simulink model "electrotac_feedback_emg"  (R2016b)
settings: Solver=FixedStepDiscrete  StartTime=0.0  StopTime=inf  FixedStep=0.02  RelTol=1e-3  EnableMultiTasking=on
undefined symbols (not defined in the file): DiscIntNeverNeededParam
libraries: PowermateLibrary x1, LIB_RehaMove3 x1, STIMYOLibrary x1
(part 1 of 3)
settings Model: SimulationMode=external  Creator=mendicus  LastModifiedBy=control
settings DataIOCC: LimitDataPoints=on  SaveFormat=Array  ReturnWorkspaceOutputs=on
settings OptimizationCC: LifeSpan=1
settings DebuggingCC: ReadBeforeWriteMsg=DisableAll  WriteAfterWriteMsg=DisableAll  WriteAfterReadMsg=DisableAll  SolverPrmCheckMsg=warning  MultiTaskDSMMsg=none  SFUnexpectedBacktrackingDiag=warning  SFNoUnconditionalDefaultTransitionDiag=warning  SFExecutionAtInitializationDiag=none
settings HardwareCC: ProdBitPerPointer=32  ProdBitPerSizeT=32  ProdBitPerPtrDiffT=32  ProdLargestAtomicFloat=None  ProdIntDivRoundTo=Undefined  ProdEndianess=Unspecified  ProdWordSize=32  ProdHWDeviceType=32-bit Generic
settings ModelReferenceCC: UpdateModelReferenceTargets=IfOutOfDate  PropagateSignalLabelsOutOfModel=off
settings SFSimCC: SFSimEcho=off
settings RTWCC: SystemTargetFile=ert_linux.tlc  MakeCommand=make_rtw OPTS=-DWITH_HW  TemplateMakefile=ert_linux.tmf  Description=Linux Embedded Coder  TargetLang=C++
settings CodeAppCC: IgnoreCustomStorageClasses=off
settings STFCustomTargetCC: ModelReferenceCompliant=off  CombineOutputUpdateFcns=on  ERTCustomFileBanners=on  SupportNonInlinedSFcns=off  RemoveResetFunc=on  SupportVariableSizeSignals=on  MATLABClassNameForMDSCustomization=Simulink.SoftwareTarget.ERTCustomization  GRTInterface=off  SystemTargetFile=ert_linux.tlc
settings ERTTargetCC: ModelReferenceCompliant=off  ParMdlRefBuildCompliant=off  CompOptLevelCompliant=off  ConcurrentExecutionCompliant=off  ERTFirstTimeCompliant=off  SupportContinuousTime=on  SupportVariableSizeSignals=on  ModelStepFunctionPrototypeControlCompliant=off  CPPClassGenCompliant=off  UseToolchainInfoCompliant=off  ExtMode=on  ERTCustomFileTemplate=ert_linux_file_process.tlc  ConvertIfToSwitch=off  SuppressUnreachableDefaultCases=off
settings ConfigComp: CovMetricSettings=dw  CovHtmlReporting=on  CovSaveCumulativeToWorkspaceVar=on  CovSaveSingleToWorkspaceVar=on  CovExternalEMLEnable=off  CovSFcnEnable=off

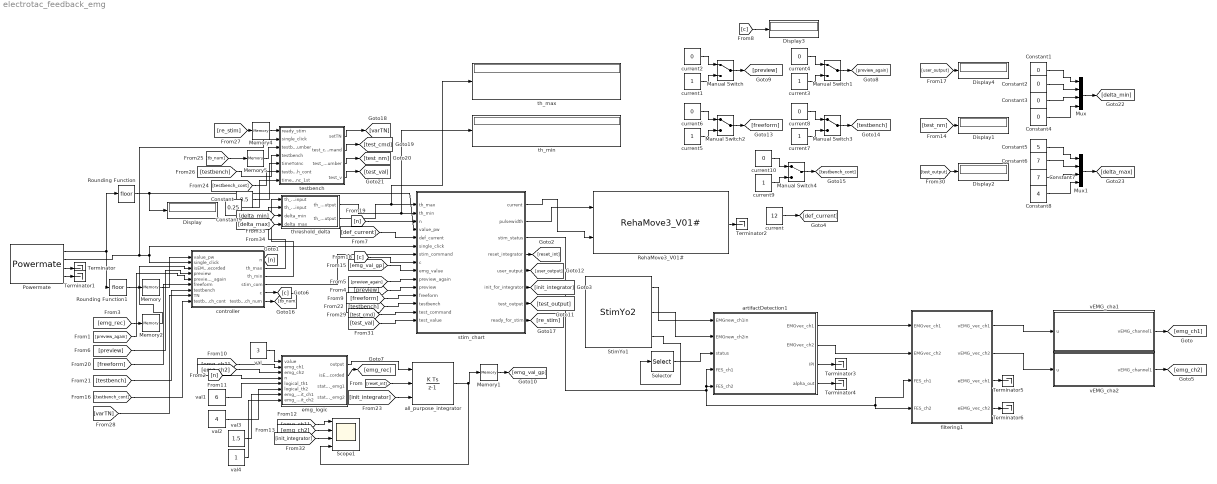
== system electrotac_feedback_emg ==
  Constant : Constant  Value=0.5
  Constant{1..4} (4 alike) : Constant  Value=0
  Constant5 : Constant  Value=5
  Constant6 : Constant  Value=7
  Constant7 : Constant  Value=7
  Constant8 : Constant  Value=4
  Constant9 : Constant  Value=0.25
  Display{,1..4} (5 alike) : Display
  Manual Switch{,1..4} (5 alike) : ManualSwitch
  Memory{,1..2,4..5} (5 alike) : Memory
  Mux : Mux
  Mux1 : Mux
  Powermate : PowermateLibrary/Powermate  pmin=0  pmax=1000  ptours=10  pstart=0  pbtnmode=0  pndoubleclick=50  Ts=0.02
  RehaMove3_V01# : LIB_RehaMove3/RehaMove3_V01#  stimDevicePath=/dev/ttyUSB0  stimChannels="[ 1  2  3  4 ]"  stimFrequency=50  stimRehaMoveProProtocol=Use the LowLevel protocol and use the user provieded pulse configs.  stimMaxCurrent=30  stimMaxPulsWidth=600  stimBlockID=STIM1  stimTextSampleTime=0.02s (based on stimulation frequency)  SampleTime=0.02  stimThreadInit=on  stimThreadData=on  stimAbortError=1  stimTestAgain=2  llPulseShape=0  llNumberOfParts=3  llMaxStimVoltage=120V  llActivateDenervation=off  mlFStim=0.5  mlFStimDynamic=off  mlFKeepAlive=1  mlUseSoftStart=off  mlUseRamps=off  mlRampsUpdates=1  mlRampsZeroUpdates=0  miscPrintBlockParam=on  miscPrintDeviceInfos=on  miscPrintSendInfos=on  miscPrintReceiveInfos=on  miscPrintInitInfos=on  miscPrintStimInfos=on  miscPrintRMPInitSettings=on  miscPrintSequenceErrors=on  miscPrintCorrectionChargeWarnings=on  miscPrintStats=on  miscUseColors=on  miscEnableAdvancedSettings=off  miscDisableVersionCheck=off
  Rounding Function : Rounding
  Rounding Function1 : Rounding
  Scope1 : Scope  NumInputPorts=4
  Selector : Selector  InputPortWidth=3  IndexOptions=Index vector (dialog)  Indices=[2]  OutputSizes=1
  StimYo1 : STIMYOLibrary/StimYo2  DeviceName='/dev/ttyUSB1'  frequency=4000  ch=[1 2]  vectorsize=200  syncmode=-1  ps_end=0  ss_start=0  ss_end=3  Ts=0.02
  Terminator{,1..6} (7 alike) : Terminator
  all_purpose_integrator : DiscreteIntegrator  ExternalReset=rising  InitialConditionSource=external  InitialConditionSetting=State (most efficient)  SampleTime=0.02  LimitOutput=on  UpperSaturationLimit=12  LowerSaturationLimit=0  ICPrevOutput=DiscIntNeverNeededParam  ICPrevScaledInput=DiscIntNeverNeededParam
  artifactDetection1 : MATLAB Function  TreatAsAtomicUnit=on  mask{emg_f_popup=4000, emg_f=4000, stim_f_popup=50, stim_f=50, L=80, peak_popup=MAD, complete=on, alpha_auto=on, alpha_init=3}
      mask prompts: emg_f_popup "EMG freq [Hz]"; emg_f "Value"; stim_f_popup "Stim freq [Hz]"; stim_f "Value"; peak_popup "Type"; complete "Last complete IPI"; alpha_auto "Automatic alpha"; alpha_init "Initial alpha"
      mask init:
      | alpha_in = [alpha_auto,alpha_init];
      | 
      | 
      | emg_ff = str2double(get_param(gcb,'emg_f'));
      | stim_ff = str2double(get_param(gcb,'stim_f'));
      | L = ceil(emg_f/stim_f);
      | assert(L <= 200, 'Maximum L = emg_f/stim_f is 200.');
  controller : Stateflow chart  TreatAsAtomicUnit=on
  current : Constant  Value=12
  current{1,3,5,7,9} (5 alike) : Constant
  current{2,4,6,8,10} (5 alike) : Constant  Value=0
  emg_logic : Stateflow chart  TreatAsAtomicUnit=on
  filtering1 : MATLAB Function  TreatAsAtomicUnit=on  mask{emg_f_popup=4000, emg_f=4000, stim_f_popup=50, stim_f=50, Tf=0.02, L=80, emg_ff=4000, stim_ff=50, vol=on, V1=20, V2=75, min_t=0.005, max_t=0.01875, evo=on, E1=20, E2=75, min_te=0.005, max_te=0.01875, peak_filter=HP filter}
      mask prompts: emg_f_popup "EMG freq [Hz]"; emg_f "Value"; stim_f_popup "Stim freq [Hz]"; stim_f "Value"; Tf "Tf [s]"; L "L [samples]"; vol "Filter volitional"; V1 "Min [samples]"; V2 "Max [samples]"; min_t "Min [s]"; max_t "Max [s]"; evo "Filter evoked"; E1 "Min [samples]"; E2 "Max [samples]"; min_te "Min [s]"; max_te "Max [s]"; peak_filter "Type"
      mask init:
      | % Test L limit
      | emg_ff = str2double(get_param(gcb,'emg_ff'));
      | stim_ff = str2double(get_param(gcb,'stim_ff'));
      | L = ceil(emg_ff/stim_ff);
      | assert(L <= 200, 'Maximum L = emg_f/stim_f is 200.');
      | 
      | % Get V1,V2 and E1,E2 (not checked)
      | maskStr_vol = get_param(gcb,'vol');
      | maskStr_evo = get_param(gcb,'evo');
      | 
      | if ~strcmp(maskStr_vol(2),'n') % check visibility
      |     V1 = 1;    V2 = 1;
      | end  
      | 
      | if ~strcmp(maskStr_evo(2),'n') % check visibility
      |     E1 = 1;    E2 = 1;
      | end
      | 
      | % Test V1,V2,E1,E2 limits
      | assert(V1 >= 1, 'Min_vol must be at least 1.');
      | assert(E1 >= 1, 'Min_evo must be at least 1.');
      | assert(V2 <= L, 'Max_vol must be lower than L.');
      | assert(E2 <= L, 'Max_evo must be lower than L.');
      | 
      | assert(V2 >= 1, 'Max_vol must be at least 1.');
      | assert(E2 >= 1, 'Max_evo must be at least 1.');
      | assert(V1 <= L, 'Min_vol must be lower than L.');
      | assert(E1 <= L, 'Min_evo must be lower than L.');
      | 
      | assert(V2 >= V1, 'Max_vol must be lower than min_vol.');
      | assert(E2 >= E1, 'Max_evo must be lower than min_evo.');
      | 
      | % Create v and e
      | v = [V1;V2];
      | e = [E1;E2];
      | 
      | % init hp filter
      | fc = 150;
      | [z,p,k] = ellip(6,3,50,fc/(emg_ff/2),'high');
      | [B,A] = zp2tf(z,p,k);
      | [F,G,E,D] = tf2ss(B,A);
      | 
      | start_emg = ceil(v(1));
      | stop_emg = ceil(v(2));
      | 
      | N = length(start_emg:stop_emg);
      | Q = eye(N)*D;
      | O = zeros(N,length(E*F));
      | emg_vol = 0;
      | for i = 1:N
      |     for j = i+1:N
      |         Q(j,i) = E*F^(j-i-1)*G;
      |     end
      |     O(i,:)=E*F^(i-1);
      | end
      | 
      | % init bp filter
      | % fc = 250;
      | % [z,p,k] = ellip(6,3,50,fc/(emg_ff/2),'high');
      | % [B,A] = zp2tf(z,p,k);
      | % [F,G,E,D] = tf2ss(B,A);
      | % 
      | % start_emg = ceil(v(1));
      | % stop_emg = ceil(v(2));
      | % 
      | % N = length(start_emg:stop_emg);
      | % Q = eye(N)*D;
      | % O = zeros(N,length(E*F));
      | % emg_vol = 0;
      | % for i = 1:N
      | %     for j = i+1:N
      | %         Q(j,i) = E*F^(j-i-1)*G;
      | %     end
      | %     O(i,:)=E*F^(i-1);
      | % end
      | 
      | EMGfilter.fc = fc;
      | EMGfilter.Q = Q;
      | EMGfilter.O = O;
      | EMGfilter.start_emg = start_emg;
      | EMGfilter.stop_emg = stop_emg;
  stim_chart : Stateflow chart  TreatAsAtomicUnit=on
  testbench : Stateflow chart  TreatAsAtomicUnit=on
  th_max : Display
  th_min : Display
  threshold_delta : MATLAB Function  TreatAsAtomicUnit=on
  vEMG_cha1 : MATLAB Function  TreatAsAtomicUnit=on
  vEMG_cha2 : MATLAB Function  TreatAsAtomicUnit=on
  val : Constant  Value=3
  val1 : Constant  Value=6
  val2 : Constant  Value=4
  val3 : Constant  Value=1.5
  val4 : Constant
  wires:
  stim_chart/2(pulsewidth) -> RehaMove3_V01#/1
  Powermate/2 -> testbench/2(single_click), stim_chart/6(single_click), controller/2(single_click)
  Powermate/1 -> Rounding Function/1, Rounding Function1/1
  Rounding Function/1 -> Display/1, stim_chart/4(value_pw)
  Rounding Function1/1 -> Memory/1
  Memory/1 -> controller/1(value_pw)
  current/1 -> [def_current]
  controller/2(th_max) -> threshold_delta/2(th_max_input)
  [def_current] -> stim_chart/5(def_current)
  controller/3(th_min) -> threshold_delta/1(th_min_input)
  controller/4(stim_com) -> stim_chart/7(stim_command)
  StimYo1/3 -> Selector/1
  StimYo1/1 -> artifactDetection1/1(EMGnew_ch1in)
  Selector/1 -> artifactDetection1/3(status)
  StimYo1/2 -> artifactDetection1/2(EMGnew_ch2in)
  stim_chart/3(stim_status) -> artifactDetection1/5(FES_ch2), artifactDetection1/4(FES_ch1), filtering1/4(FES_ch2), filtering1/3(FES_ch1)
  artifactDetection1/1(EMGvec_ch1) -> filtering1/1(EMGvec_ch1)
  artifactDetection1/2(EMGvec_ch2) -> filtering1/2(EMGvec_ch2)
  Powermate/3 -> Terminator/1
  Powermate/4 -> Terminator1/1
  RehaMove3_V01#/1 -> Terminator2/1
  artifactDetection1/3(IPI) -> Terminator3/1
  stim_chart/1(current) -> RehaMove3_V01#/2
  artifactDetection1/4(alpha_out) -> Terminator4/1
  filtering1/3(eEMG_vec_ch1) -> Terminator5/1
  filtering1/4(eEMG_vec_ch2) -> Terminator6/1
  filtering1/2(vEMG_vec_ch2) -> vEMG_cha2/1(u)
  emg_logic/1(output) -> all_purpose_integrator/1
  val/1 -> emg_logic/1(value)
  [emg_ch2] -> emg_logic/3(emg_ch2)
  [emg_ch1] -> emg_logic/2(emg_ch1)
  stim_chart/4(reset_integrator) -> [reset_int]
  [reset_int] -> all_purpose_integrator/2
  controller/1(n) -> [n]
  [n] -> emg_logic/4(n)
  emg_logic/2(isEMGrecorded) -> [emg_rec]
  val1/1 -> emg_logic/5(logical_th1)
  val2/1 -> emg_logic/6(logical_th2)
  filtering1/1(vEMG_vec_ch1) -> vEMG_cha1/1(u)
  vEMG_cha1/1(vEMG_channel1) -> [emg_ch1]
  vEMG_cha2/1(vEMG_channel1) -> [emg_ch2]
  [emg_rec] -> Memory2/1
  Memory2/1 -> controller/3(isEMGrecorded)
  current2/1 -> Manual Switch/1
  controller/5(c) -> [c]
  [preview] -> stim_chart/11(preview)
  [preview_again] -> stim_chart/10(preview_again)
  [preview_again] -> controller/5(preview_again)
  [preview] -> controller/4(preview)
  [c] -> Display3/1
  [emg_ch1] -> Scope1/1
  [emg_ch2] -> Scope1/2
  Memory1/1 -> [emg_val_gp]
  [emg_val_gp] -> stim_chart/9(emg_value)
  stim_chart/5(user_output) -> [user_output]
  [user_output] -> Display4/1
  [c] -> stim_chart/8(c)
  [n] -> stim_chart/3(n)
  current1/1 -> Manual Switch/2
  Manual Switch/1 -> [preview]
  current4/1 -> Manual Switch1/1
  current3/1 -> Manual Switch1/2
  Manual Switch1/1 -> [preview_again]
  current6/1 -> Manual Switch2/1
  current5/1 -> Manual Switch2/2
  Manual Switch2/1 -> [freeform]
  current8/1 -> Manual Switch3/1
  current7/1 -> Manual Switch3/2
  Manual Switch3/1 -> [testbench]
  controller/6(testbench_num) -> [tb_num]
  [freeform] -> controller/6(freeform)
  [testbench] -> controller/7(testbench)
  [freeform] -> stim_chart/12(freeform)
  [testbench] -> stim_chart/13(testbench)
  stim_chart/6(init_for_integrator) -> [init_integrator]
  [init_integrator] -> all_purpose_integrator/3
  stim_chart/7(test_output) -> [test_output]
  [tb_num] -> Memory5/1
  [testbench] -> testbench/4(testbench)
  stim_chart/8(ready_for_stim) -> [re_stim]
  testbench/1(setTN) -> [varTN]
  [varTN] -> controller/8(TN)
  testbench/2(test_command) -> [test_cmd]
  testbench/3(test_number) -> [test_nm]
  [test_cmd] -> stim_chart/14(test_command)
  testbench/4(test_v) -> [test_val]
  [test_val] -> stim_chart/15(test_value)
  [re_stim] -> Memory4/1
  Memory4/1 -> testbench/1(ready_stim)
  Memory5/1 -> testbench/3(testbench_number)
  [test_output] -> Display2/1
  [init_integrator] -> Scope1/3
  all_purpose_integrator/1 -> Scope1/4, Memory1/1
  [test_nm] -> Display1/1
  [testbench_cont] -> controller/9(testbench_cont)
  [testbench_cont] -> testbench/6(testbench_cont)
  current10/1 -> Manual Switch4/1
  current9/1 -> Manual Switch4/2
  Manual Switch4/1 -> [testbench_cont]
  Constant/1 -> testbench/5(timeToInc)
  threshold_delta/1(th_min_output) -> th_min/1, stim_chart/2(th_min)
  threshold_delta/2(th_max_output) -> th_max/1, stim_chart/1(th_max)
  [delta_min] -> threshold_delta/3(delta_min)
  [delta_max] -> threshold_delta/4(delta_max)
  Constant1/1 -> Mux/1
  Constant2/1 -> Mux/2
  Constant3/1 -> Mux/3
  Constant4/1 -> Mux/4
  Mux/1 -> [delta_min]
  Constant5/1 -> Mux1/1
  Constant6/1 -> Mux1/2
  Constant7/1 -> Mux1/3
  Constant8/1 -> Mux1/4
  Mux1/1 -> [delta_max]
  val3/1 -> emg_logic/7(emg_limit_ch1)
  val4/1 -> emg_logic/8(emg_limit_ch2)
  Constant9/1 -> testbench/7(timeToInc_1st)

== stateflow chart electrotac_feedback_emg/controller ==
  state init
    entry:
    th_min = [0 0 0 0];
    th_max = [0 0 0 0];
  state ch1_max1/
    entry:
    n = 2
    exit:
    max_e1 = value_pw;
  state dummy1
  state ch1_min/
    entry:
    n = 1
    exit:
    min_e1 = value_pw;
  state dummy
  state dummy2
  state ch1_min1/
    entry:
    n = 3
    exit:
    min_e2 = value_pw;
  state ch1_max2/
    entry:
    n = 4
    exit:
    max_e2 = value_pw;
  state dummy3
  state dummy4
  state ch2_min1/
    entry:
    n = 5
    exit:
    min_e3 = value_pw;
  state ch2_max1/
    entry:
    n = 6
    exit:
    max_e3 = value_pw;
  state dummy5
  state dummy6
  state ch2_min2/
    entry:
    n = 7
    exit:
    min_e4 = value_pw;
  state dummy7
  state ch2_max2/
    entry:
    n = 8
    exit:
    max_e4 = value_pw;
  state dummy8
  state results/
    entry:
    n = 9
    th_min = [min_e1, min_e2, min_e3, min_e4];
    th_max = [max_e1, max_e2, max_e3, max_e4];
  state emg_ch1
    entry:
  state dummy9
    entry: n = 10
  state dummy10
  state emg_ch2
    entry: n = 11;
  state testsuite
    state output_Rand
      entry:
      testbench_num = rand_vec(counter);
    state generate_rand_vec
      entry:
      counter = 1;
      rand_vec = randperm(5);
      testbench_num = 0;
    state dummy
    state selector
    state dummy1
    state counter_eq10
    state delay
    testsuite.output_Rand -> testsuite.selector : [single_click == 1 && TN == 1]{counter = counter + 1;}
    testsuite.dummy -> testsuite.output_Rand : after(1,sec)
    (default) -> generate_rand_vec
    generate_rand_vec -> testsuite.dummy : [single_click == 1 && TN == 1]
    testsuite.selector -> testsuite.dummy [order 2] : [counter ~= 6]
    testsuite.selector -> testsuite.delay [order 1] : [counter == 6]
    testsuite.dummy1 -> generate_rand_vec : after(1,sec)
    testsuite.counter_eq10 -> testsuite.dummy1 : [single_click == 1]
    testsuite.delay -> testsuite.counter_eq10 : after(1,sec)
  state testsuite_cont
    state output_Rand
      entry:
      testbench_num = rand_vec2(counter);
    state generate_rand_vec1
      entry:
      counter = 1;
      rand_vec2 = randperm(3);
      testbench_num = 0;
    state dummy12
    state selector
    state dummy11
    state counter_eq10
    state delay
    testsuite_cont.output_Rand -> testsuite_cont.selector : [single_click == 1 && TN == 1]{counter = counter + 1;}
    dummy12 -> testsuite_cont.output_Rand : after(1,sec)
    (default) -> generate_rand_vec1
    generate_rand_vec1 -> dummy12 : [single_click == 1 && TN == 1]
    testsuite_cont.selector -> dummy12 [order 2] : [counter ~= 4]
    testsuite_cont.selector -> testsuite_cont.delay [order 1] : [counter == 4]
    dummy11 -> generate_rand_vec1 : after(1,sec)
    testsuite_cont.counter_eq10 -> dummy11 : [single_click == 1]
    testsuite_cont.delay -> testsuite_cont.counter_eq10 : after(1,sec)
  state change_n
    entry: n = 12;
  state preview_changer
    entry: c = 0;
    state wait_for_command
    state change_state
      entry: c = c + 1;
    state limit_reached
    state NOP
    (default) -> preview_changer.wait_for_command
    preview_changer.wait_for_command -> preview_changer.change_state : [single_click == 1]
    preview_changer.change_state -> preview_changer.limit_reached [order 2] : [c == 28]
    preview_changer.change_state -> preview_changer.wait_for_command [order 1] : after(1,sec)
    preview_changer.NOP -> preview_changer.wait_for_command : [preview_again == 1]{c = 0}
    preview_changer.limit_reached -> preview_changer.NOP : after(1,sec)
  state freeform_changer
    entry: stim_com = 0;
    state wait_for_command
    state change_state
      entry: stim_com = stim_com + 1;
    state limit_reached
    state NOP
    state reset_stimcom
      entry:
      stim_com = 1;
    (default) -> freeform_changer.wait_for_command
    freeform_changer.wait_for_command -> freeform_changer.change_state : [single_click == 1]
    freeform_changer.change_state -> freeform_changer.limit_reached [order 2] : [stim_com == 4]
    freeform_changer.change_state -> freeform_changer.wait_for_command [order 1] : after(1,sec)
    reset_stimcom -> freeform_changer.wait_for_command : after(1,sec)
    freeform_changer.NOP -> reset_stimcom : [single_click == 1]
    freeform_changer.limit_reached -> freeform_changer.NOP : after(1,sec)
  (default) -> init
  ch1_min -> dummy1 : [single_click == 1]
  dummy1 -> ch1_max1 : after(1,sec)
  dummy -> ch1_min : after(1,sec)
  init -> dummy : [single_click == 1]
  ch1_max1 -> dummy2 : [single_click == 1]
  dummy2 -> ch1_min1 : after(1,sec)
  ch1_min1 -> dummy3 : [single_click == 1]
  dummy3 -> ch1_max2 : after(1,sec)
  ch1_max2 -> dummy4 : [single_click == 1]
  dummy4 -> ch2_min1 : after(1,sec)
  ch2_min1 -> dummy5 : [single_click == 1]
  dummy5 -> ch2_max1 : after(1,sec)
  ch2_max1 -> dummy6 : [single_click == 1]
  dummy6 -> ch2_min2 : after(1,sec)
  ch2_min2 -> dummy7 : [single_click == 1]
  dummy7 -> ch2_max2 : after(1,sec)
  ch2_max2 -> results : [single_click == 1]
  results -> dummy8 : after(1,sec)
  dummy8 -> emg_ch1 : [isEMGrecorded == 0]
  emg_ch1 -> dummy9 : [isEMGrecorded== 1]
  dummy9 -> dummy10 : [isEMGrecorded == 0]
  dummy10 -> emg_ch2 : after(1,sec)
  emg_ch2 -> change_n : [isEMGrecorded == 1]
  change_n -> testsuite [order 3] : [testbench == 1]
  testsuite -> change_n [order 1] : [testbench == 0]
  change_n -> freeform_changer [order 2] : [freeform == 1]
  testsuite -> testsuite_cont [order 2] : [testbench_cont == 1]
  freeform_changer -> change_n : [freeform == 0]
  testsuite_cont -> testsuite : [testbench_cont ~= 1]
  change_n -> preview_changer [order 1] : [preview == 1]
  preview_changer -> change_n : [preview == 0]
  data: value_pw input; single_click input; n output; th_max output size=[1 4]; th_min output size=[1 4]; min_e2 local; min_e1 local; max_e2 local; max_e1 local; max_e3 local; min_e3 local; min_e4 local; max_e4 local; stim_com output; isEMGrecorded input; preview input; preview_again input; c output; freeform input; counter local; rand_vec local; testbench input; testbench_num output; TN input; testbench_cont input; rand_vec2 local

== stateflow chart electrotac_feedback_emg/testbench ==
  state init_for_cont
    state tes_cont1
      % hand from 0 to 90 to 135 to 0
      entry: setTN = 0;
      state hand_to_270d
        entry: test_v = 0;
        state increment
          entry: test_v = test_v + 0.5;
        state cmd
          entry:
        state wait
        (default) -> init_for_cont.tes_cont1.hand_to_270d.increment
        init_for_cont.tes_cont1.hand_to_270d.increment -> init_for_cont.tes_cont1.hand_to_270d.wait : after(timeToInc_1st,sec)
        init_for_cont.tes_cont1.hand_to_270d.wait -> init_for_cont.tes_cont1.hand_to_270d.increment [order 2] : after(timeToInc,sec)
        init_for_cont.tes_cont1.hand_to_270d.wait -> init_for_cont.tes_cont1.hand_to_270d.cmd [order 1] : [test_v == 3]
      state close_hand1
        entry: test_v = 3;
        state increment
          entry: test_v = test_v + 0.5;
        state cmd
          entry:
        state wait
        (default) -> init_for_cont.tes_cont1.close_hand1.increment
        init_for_cont.tes_cont1.close_hand1.increment -> init_for_cont.tes_cont1.close_hand1.wait : after(timeToInc_1st,sec)
        init_for_cont.tes_cont1.close_hand1.wait -> init_for_cont.tes_cont1.close_hand1.increment [order 2] : after(timeToInc,sec)
        init_for_cont.tes_cont1.close_hand1.wait -> init_for_cont.tes_cont1.close_hand1.cmd [order 1] : [test_v == 4.5]
      state foo
        entry: test_v = 4.5;
        state increment
          entry: test_v = test_v  - 0.5;
        state cmd
          entry:
          setTN = 1;
        state wait
        (default) -> init_for_cont.tes_cont1.foo.increment
        init_for_cont.tes_cont1.foo.increment -> init_for_cont.tes_cont1.foo.wait : after(timeToInc_1st,sec)
        init_for_cont.tes_cont1.foo.wait -> init_for_cont.tes_cont1.foo.increment [order 2] : after(timeToInc,sec)
        init_for_cont.tes_cont1.foo.wait -> init_for_cont.tes_cont1.foo.cmd [order 1] : after(0.5,sec)[test_v == 0]
      state start_test1
        entry:
        test_number = 8010;
      state hand
        entry:
        test_command = 4;
        test_number = 8011;
      state opcl
        entry:
        test_command = 4;
        test_number = 8012;
      state force0c5
        entry:
        test_command = 4;
        test_number = 8013;
      (default) -> init_for_cont.tes_cont1.start_test1
      init_for_cont.tes_cont1.start_test1 -> init_for_cont.tes_cont1.hand : [single_click == 1]
      init_for_cont.tes_cont1.hand -> init_for_cont.tes_cont1.hand_to_270d : [ready_stim == 1]
      init_for_cont.tes_cont1.hand_to_270d.cmd -> init_for_cont.tes_cont1.opcl : [single_click == 1]
      init_for_cont.tes_cont1.opcl -> init_for_cont.tes_cont1.close_hand1 : [ready_stim == 1]
      init_for_cont.tes_cont1.force0c5 -> init_for_cont.tes_cont1.foo : [ready_stim == 1]
      init_for_cont.tes_cont1.close_hand1.cmd -> init_for_cont.tes_cont1.force0c5 : [single_click == 1]
    state tes_cont2
      % hand from 315 to 90 to 270 to 0
      entry: setTN = 0;
      state hand_to_270d
        entry: test_v = 10.5;
        state increment
          entry: test_v = test_v - 0.5;
        state cmd
          entry:
        state wait
        (default) -> init_for_cont.tes_cont2.hand_to_270d.increment
        init_for_cont.tes_cont2.hand_to_270d.increment -> init_for_cont.tes_cont2.hand_to_270d.wait : after(timeToInc_1st,sec)
        init_for_cont.tes_cont2.hand_to_270d.wait -> init_for_cont.tes_cont2.hand_to_270d.increment [order 2] : after(timeToInc,sec)
        init_for_cont.tes_cont2.hand_to_270d.wait -> init_for_cont.tes_cont2.hand_to_270d.cmd [order 1] : [test_v == 3]
      state close_hand1
        entry: test_v = 3;
        state increment
          entry: test_v = test_v + 0.5;
        state cmd
          entry:
        state wait
        (default) -> init_for_cont.tes_cont2.close_hand1.increment
        init_for_cont.tes_cont2.close_hand1.increment -> init_for_cont.tes_cont2.close_hand1.wait : after(timeToInc_1st,sec)
        init_for_cont.tes_cont2.close_hand1.wait -> init_for_cont.tes_cont2.close_hand1.increment [order 2] : after(timeToInc,sec)
        init_for_cont.tes_cont2.close_hand1.wait -> init_for_cont.tes_cont2.close_hand1.cmd [order 1] : [test_v == 9]
      state foo
        entry: test_v = 9;
        state increment
          entry: test_v = test_v - 0.5;
        state cmd
          entry:
          setTN = 1;
        state wait
        (default) -> init_for_cont.tes_cont2.foo.increment
        init_for_cont.tes_cont2.foo.increment -> init_for_cont.tes_cont2.foo.wait : after(timeToInc_1st,sec)
        init_for_cont.tes_cont2.foo.wait -> init_for_cont.tes_cont2.foo.increment [order 2] : after(timeToInc,sec)
        init_for_cont.tes_cont2.foo.wait -> init_for_cont.tes_cont2.foo.cmd [order 1] : after(0.5,sec)[test_v == 0]
      state start_test1
        entry:
        test_number = 8020;
      state hand
        entry:
        test_command = 4;
        test_number = 8021;
      state opcl
        entry:
        test_command = 4;
        test_number = 8022;
      state force0c5
        entry:
        test_command = 4;
        test_number = 8023;
      (default) -> init_for_cont.tes_cont2.start_test1
      init_for_cont.tes_cont2.start_test1 -> init_for_cont.tes_cont2.hand : [single_click == 1]
      init_for_cont.tes_cont2.hand -> init_for_cont.tes_cont2.hand_to_270d : [ready_stim == 1]
      init_for_cont.tes_cont2.hand_to_270d.cmd -> init_for_cont.tes_cont2.opcl : [single_click == 1]
      init_for_cont.tes_cont2.opcl -> init_for_cont.tes_cont2.close_hand1 : [ready_stim == 1]
      init_for_cont.tes_cont2.force0c5 -> init_for_cont.tes_cont2.foo : [ready_stim == 1]
      init_for_cont.tes_cont2.close_hand1.cmd -> init_for_cont.tes_cont2.force0c5 : [single_click == 1]
    state start_
      entry: setTN = 1;
      test_number = 8888;
    state waitForInput2
      entry: test_command = 0;
    state tes_cont3
      % hand from 120 to 30 to 225 to 0
      entry: setTN = 0;
      state hand_to_270d
        entry: test_v = 4;
        state increment
          entry: test_v = test_v - 0.5;
        state cmd
          entry:
        state wait
        (default) -> init_for_cont.tes_cont3.hand_to_270d.increment
        init_for_cont.tes_cont3.hand_to_270d.increment -> init_for_cont.tes_cont3.hand_to_270d.wait : after(timeToInc_1st,sec)
        init_for_cont.tes_cont3.hand_to_270d.wait -> init_for_cont.tes_cont3.hand_to_270d.increment [order 2] : after(timeToInc,sec)
        init_for_cont.tes_cont3.hand_to_270d.wait -> init_for_cont.tes_cont3.hand_to_270d.cmd [order 1] : [test_v == 1]
      state close_hand1
        entry: test_v = 1;
        state increment
          entry: test_v = test_v + 0.5;
        state cmd
          entry:
        state wait
        (default) -> init_for_cont.tes_cont3.close_hand1.increment
        init_for_cont.tes_cont3.close_hand1.increment -> init_for_cont.tes_cont3.close_hand1.wait : after(timeToInc_1st,sec)
        init_for_cont.tes_cont3.close_hand1.wait -> init_for_cont.tes_cont3.close_hand1.increment [order 2] : after(timeToInc,sec)
        init_for_cont.tes_cont3.close_hand1.wait -> init_for_cont.tes_cont3.close_hand1.cmd [order 1] : [test_v == 7.5]
      state foo
        entry: test_v = 7.5;
        state increment
          entry: test_v = test_v - 0.5;
        state cmd
          entry:
          setTN = 1;
        state wait
        (default) -> init_for_cont.tes_cont3.foo.increment
        init_for_cont.tes_cont3.foo.increment -> init_for_cont.tes_cont3.foo.wait : after(timeToInc_1st,sec)
        init_for_cont.tes_cont3.foo.wait -> init_for_cont.tes_cont3.foo.increment [order 2] : after(timeToInc,sec)
        init_for_cont.tes_cont3.foo.wait -> init_for_cont.tes_cont3.foo.cmd [order 1] : after(0.5,sec)[test_v == 0]
      state start_test1
        entry:
        test_number = 8030;
      state hand
        entry:
        test_command = 4;
        test_number = 8031;
      state opcl
        entry:
        test_command = 4;
        test_number = 8032;
      state force0c5
        entry:
        test_command = 4;
        test_number = 8033;
      (default) -> init_for_cont.tes_cont3.start_test1
      init_for_cont.tes_cont3.start_test1 -> init_for_cont.tes_cont3.hand : [single_click == 1]
      init_for_cont.tes_cont3.hand -> init_for_cont.tes_cont3.hand_to_270d : [ready_stim == 1]
      init_for_cont.tes_cont3.hand_to_270d.cmd -> init_for_cont.tes_cont3.opcl : [single_click == 1]
      init_for_cont.tes_cont3.opcl -> init_for_cont.tes_cont3.close_hand1 : [ready_stim == 1]
      init_for_cont.tes_cont3.force0c5 -> init_for_cont.tes_cont3.foo : [ready_stim == 1]
      init_for_cont.tes_cont3.close_hand1.cmd -> init_for_cont.tes_cont3.force0c5 : [single_click == 1]
    tes_cont1 -> start_ : [testbench_number ~= 1]
    waitForInput2 -> tes_cont1 [order 1] : [testbench_number == 1]
    (default) -> start_
    waitForInput2 -> tes_cont2 [order 2] : [testbench_number == 2]
    start_ -> waitForInput2 : after(0.5,sec)
    waitForInput2 -> tes_cont3 [order 3] : [testbench_number == 3]
    tes_cont2 -> start_ : [testbench_number ~= 2]
    tes_cont3 -> start_ : [testbench_number ~= 3]
  state template [group] [commented out]
    state force1_to_force0 [commented out]
      entry: test_v = 0;
      state increment [commented out]
        entry: test_v = test_v + 1;
      state wait1 [commented out]
      state cmd [commented out]
        entry:
        test_number = 9032;
        setTN = 1;
      state wait [commented out]
      state decrement [commented out]
        entry: test_v = test_v - 1;
      template.force1_to_force0.wait1 -> template.force1_to_force0.cmd [commented out] : [test_v == 0]
      (default) -> template.force1_to_force0.increment [commented out]
      template.force1_to_force0.wait1 -> template.force1_to_force0.decrement [commented out] : after(timeToInc,sec)
      template.force1_to_force0.decrement -> template.force1_to_force0.wait1 [commented out]
      template.force1_to_force0.increment -> template.force1_to_force0.wait [commented out]
      template.force1_to_force0.wait -> template.force1_to_force0.increment [commented out] : after(timeToInc,sec)
      template.force1_to_force0.wait -> template.force1_to_force0.decrement [commented out] : [test_v == 7]
    state opcl2 [commented out]
      entry:
      test_command = 2;
    (default) -> template.opcl2 [commented out] : [single_click == 1]
    template.opcl2 -> template.force1_to_force0 [commented out] : [ready_stim == 1]
  state test1
    % turn hand to 270 degrees -> close the hand -> force 0.5
    entry: setTN = 0;
    state hand_to_270d
      entry: test_v = 0;
      state increment
        entry: test_v = test_v + 1;
      state cmd
        entry:
      state wait
      (default) -> test1.hand_to_270d.increment
      test1.hand_to_270d.increment -> test1.hand_to_270d.wait : after(timeToInc_1st,sec)
      test1.hand_to_270d.wait -> test1.hand_to_270d.increment [order 2] : after(timeToInc,sec)
      test1.hand_to_270d.wait -> test1.hand_to_270d.cmd [order 1] : [test_v == 10]
    state close_hand1
      entry: test_v = 0;
      state increment
        entry: test_v = test_v + 1;
      state cmd
        entry:
      state wait
      (default) -> test1.close_hand1.increment
      test1.close_hand1.increment -> test1.close_hand1.wait : after(timeToInc_1st,sec)
      test1.close_hand1.wait -> test1.close_hand1.increment [order 2] : after(timeToInc,sec)
      test1.close_hand1.wait -> test1.close_hand1.cmd [order 1] : [test_v == 12]
    state foo
      entry: test_v = 0;
      state increment
        entry: test_v = test_v + 1;
      state cmd
        entry:
        setTN = 1;
      state wait
      (default) -> test1.foo.increment
      test1.foo.increment -> test1.foo.wait : after(timeToInc_1st,sec)
      test1.foo.wait -> test1.foo.increment [order 2] : after(timeToInc,sec)
      test1.foo.wait -> test1.foo.cmd [order 1] : after(0.5,sec)[test_v == 6]
    state start_test1
      entry:
      test_number = 9010;
    state hand
      entry:
      test_command = 1;
      test_number = 9011;
    state opcl
      entry:
      test_command = 2;
      test_number = 9012;
    state force0c5
      entry:
      test_command = 3;
      test_number = 9013;
    (default) -> test1.start_test1
    test1.start_test1 -> test1.hand : [single_click == 1]
    test1.hand -> test1.hand_to_270d : [ready_stim == 1]
    test1.hand_to_270d.cmd -> test1.opcl : [single_click == 1]
    test1.opcl -> test1.close_hand1 : [ready_stim == 1]
    test1.force0c5 -> test1.foo : [ready_stim == 1]
    test1.close_hand1.cmd -> test1.force0c5 : [single_click == 1]
  state template2 [group] [commented out]
    state hand_to_270d [commented out]
      entry: test_v = 12;
      state increment [commented out]
        entry: test_v = test_v - 1;
      state cmd [commented out]
        entry:
        test_number = 9031;
      state wait [commented out]
      (default) -> template2.hand_to_270d.increment [commented out]
      template2.hand_to_270d.increment -> template2.hand_to_270d.wait [commented out]
      template2.hand_to_270d.wait -> template2.hand_to_270d.increment [commented out] : after(timeToInc,sec)
      template2.hand_to_270d.wait -> template2.hand_to_270d.cmd [commented out] : [test_v == 4]
    state opcl1 [commented out]
      entry:
      test_command = 2;
    template2.opcl1 -> template2.hand_to_270d [commented out] : [ready_stim == 1]
    template2.hand_to_270d.cmd -> ? [commented out] : [single_click == 1]
  state start
    entry:
    setTN = 1;
    test_number = 9999;
  state test2
    %close the hand -> force 1 -> force 0.25 -> open the hand
    entry: setTN = 0;
    state hand_to_270d
      entry: test_v = 0;
      state increment
        entry: test_v = test_v + 1;
      state cmd
        entry:
      state wait
      (default) -> test2.hand_to_270d.increment
      test2.hand_to_270d.increment -> test2.hand_to_270d.wait : after(timeToInc_1st,sec)
      test2.hand_to_270d.wait -> test2.hand_to_270d.increment [order 2] : after(timeToInc,sec)
      test2.hand_to_270d.wait -> test2.hand_to_270d.cmd [order 1] : [test_v == 12]
    state force1_to_force0
      entry: test_v = 0;
      state increment
        entry: test_v = test_v + 1;
      state wait1
      state cmd
        entry:
      state wait
      state decrement
        entry: test_v = test_v - 1;
      (default) -> test2.force1_to_force0.increment
      test2.force1_to_force0.wait1 -> test2.force1_to_force0.cmd [order 1] : [test_v == 3]
      test2.force1_to_force0.wait1 -> test2.force1_to_force0.decrement [order 2] : after(timeToInc,sec)
      test2.force1_to_force0.decrement -> test2.force1_to_force0.wait1
      test2.force1_to_force0.increment -> test2.force1_to_force0.wait : after(timeToInc_1st,sec)
      test2.force1_to_force0.wait -> test2.force1_to_force0.increment [order 2] : after(timeToInc,sec)
      test2.force1_to_force0.wait -> test2.force1_to_force0.decrement [order 1] : [test_v == 12]
    state foo
      entry: test_v = 12;
      state increment
        entry: test_v = test_v - 1;
      state cmd
        entry:
        setTN = 1;
      state wait
      (default) -> test2.foo.increment
      test2.foo.increment -> test2.foo.wait : after(timeToInc_1st,sec)
      test2.foo.wait -> test2.foo.increment [order 2] : after(timeToInc,sec)
      test2.foo.wait -> test2.foo.cmd [order 1] : after(0.5,sec)[test_v == 0]
    state start_test1
      entry:
      test_number = 9020;
    state opcl1
      entry:
      test_command = 2;
      test_number = 9021;
    state opcl
      entry:
      test_command = 3;
      test_number = 9022;
    state force0c5
      entry:
      test_command = 2;
      test_number = 9023;
    (default) -> test2.start_test1
    test2.start_test1 -> test2.opcl1 : [single_click == 1]
    test2.opcl1 -> test2.hand_to_270d : [ready_stim == 1]
    test2.hand_to_270d.cmd -> test2.opcl : [single_click == 1]
    test2.opcl -> test2.force1_to_force0 : [ready_stim == 1]
    test2.force0c5 -> test2.foo : [ready_stim == 1]
    test2.force1_to_force0.cmd -> test2.force0c5 : [single_click == 1]
  state init
  state waitForInput1
    entry: test_command = 0;
  state test3
    %hand 360 to 90 -> close hand - level 2 > force 1 > open the hand
    entry: setTN = 0;
    state hand_to_270d
      entry: test_v = 12;
      state increment
        entry: test_v = test_v - 1;
      state cmd
        entry:
      state wait
      (default) -> test3.hand_to_270d.increment
      test3.hand_to_270d.increment -> test3.hand_to_270d.wait : after(timeToInc_1st,sec)
      test3.hand_to_270d.wait -> test3.hand_to_270d.increment [order 2] : after(timeToInc,sec)
      test3.hand_to_270d.wait -> test3.hand_to_270d.cmd [order 1] : [test_v == 4]
    state hand_to_270d2
      entry: test_v = 0;
      state increment
        entry: test_v = test_v + 1;
      state cmd
        entry:
      state wait
      (default) -> test3.hand_to_270d2.increment
      test3.hand_to_270d2.increment -> test3.hand_to_270d2.wait : after(timeToInc_1st,sec)
      test3.hand_to_270d2.wait -> test3.hand_to_270d2.increment [order 2] : after(timeToInc,sec)
      test3.hand_to_270d2.wait -> test3.hand_to_270d2.cmd [order 1] : [test_v == 12]
    state hand_to_270d1
      entry: test_v = 0;
      state increment
        entry: test_v = test_v + 1;
      state cmd
        entry:
      state wait
      (default) -> test3.hand_to_270d1.increment
      test3.hand_to_270d1.increment -> test3.hand_to_270d1.wait : after(timeToInc_1st,sec)
      test3.hand_to_270d1.wait -> test3.hand_to_270d1.increment [order 2] : after(timeToInc,sec)
      test3.hand_to_270d1.wait -> test3.hand_to_270d1.cmd [order 1] : [test_v == 7]
    state hand_to_270d3
      entry: test_v = 7;
      state increment
        entry: test_v = test_v - 1;
      state cmd
        entry:
        setTN = 1;
      state wait
      (default) -> test3.hand_to_270d3.increment
      test3.hand_to_270d3.increment -> test3.hand_to_270d3.wait : after(timeToInc_1st,sec)
      test3.hand_to_270d3.wait -> test3.hand_to_270d3.increment [order 2] : after(timeToInc,sec)
      test3.hand_to_270d3.wait -> test3.hand_to_270d3.cmd [order 1] : after(0.5,sec)[test_v == 0]
    state start_test1
      entry:
      test_number = 9030;
    state opcl1
      entry:
      test_command = 1;
      test_number = 9031;
    state opcl
      entry:
      test_command = 2;
      test_number = 9032;
    state opcl2
      entry:
      test_command = 3;
      test_number = 9033;
    state opcl3
      entry:
      test_command = 2;
      test_number = 9034;
    (default) -> test3.start_test1
    test3.start_test1 -> test3.opcl1 : [single_click == 1]
    test3.opcl1 -> test3.hand_to_270d : [ready_stim == 1]
    test3.opcl2 -> hand_to_270d2 : [ready_stim == 1]
    test3.opcl3 -> hand_to_270d3 : [ready_stim == 1]
    test3.hand_to_270d.cmd -> test3.opcl : [single_click == 1]
    test3.hand_to_270d2.cmd -> test3.opcl3 : [single_click == 1]
    test3.hand_to_270d1.cmd -> test3.opcl2 : [single_click == 1]
    test3.opcl -> hand_to_270d1 : [ready_stim == 1]
  state test4
    % close hand level 1 - hand to 135 - force 0.75 - hand to 225
    entry: setTN = 0;
    state hand_to_270d
      entry: test_v = 0;
      state increment
        entry: test_v = test_v + 1;
      state cmd
        entry:
      state wait
      (default) -> test4.hand_to_270d.increment
      test4.hand_to_270d.increment -> test4.hand_to_270d.wait : after(timeToInc_1st,sec)
      test4.hand_to_270d.wait -> test4.hand_to_270d.increment [order 2] : after(timeToInc,sec)
      test4.hand_to_270d.wait -> test4.hand_to_270d.cmd [order 1] : [test_v == 4]
    state force1_to_force0
      entry: test_v = 0;
      state increment
        entry: test_v = test_v + 1;
      state cmd
        entry:
      state wait
      (default) -> test4.force1_to_force0.increment
      test4.force1_to_force0.wait -> test4.force1_to_force0.cmd [order 1] : [test_v == 5]
      test4.force1_to_force0.increment -> test4.force1_to_force0.wait : after(timeToInc_1st,sec)
      test4.force1_to_force0.wait -> test4.force1_to_force0.increment [order 2] : after(timeToInc,sec)
    state hand_dto_270d
      entry: test_v = 0;
      state increment
        entry: test_v = test_v + 1;
      state cmd
        entry:
      state wait
      (default) -> test4.hand_dto_270d.increment
      test4.hand_dto_270d.increment -> test4.hand_dto_270d.wait : after(timeToInc_1st,sec)
      test4.hand_dto_270d.wait -> test4.hand_dto_270d.increment [order 2] : after(timeToInc,sec)
      test4.hand_dto_270d.wait -> test4.hand_dto_270d.cmd [order 1] : [test_v == 9]
    state haand_to_270d
      entry: test_v = 0;
      state increment
        entry: test_v = test_v + 1;
      state cmd
        entry:
        setTN = 1;
      state wait
      (default) -> test4.haand_to_270d.increment
      test4.haand_to_270d.increment -> test4.haand_to_270d.wait : after(timeToInc_1st,sec)
      test4.haand_to_270d.wait -> test4.haand_to_270d.increment [order 2] : after(timeToInc,sec)
      test4.haand_to_270d.wait -> test4.haand_to_270d.cmd [order 1] : after(0.5,sec)[test_v == 8]
    state opcl2
      entry:
      test_command = 3;
      test_number = 9043;
    state start_test1
      entry:
      test_number = 9040;
    state opcl1
      entry:
      test_command = 2;
      test_number = 9041;
    state opcl
      entry:
      test_command = 1;
      test_number = 9042;
    state opcl3
      entry:
      test_command = 1;
      test_number = 9044;
    (default) -> test4.start_test1
    test4.start_test1 -> test4.opcl1 : [single_click == 1]
    test4.opcl2 -> test4.hand_dto_270d : [ready_stim == 1]
    test4.force1_to_force0 -> test4.opcl2 : [single_click == 1]
    test4.opcl1 -> test4.hand_to_270d : [ready_stim == 1]
    test4.opcl3 -> test4.haand_to_270d : [ready_stim == 1]
    test4.hand_to_270d.cmd -> test4.opcl : [single_click == 1]
    test4.opcl -> test4.force1_to_force0 : [ready_stim == 1]
    test4.hand_dto_270d.cmd -> test4.opcl3 : [single_click == 1]
  state test5
    % force 1 to 0.5 -> turn hand 225 to 45 -> open hand 3 to 1
    % hand 45 to 135
    entry: setTN = 0;
    state hand_to_270d
      entry: test_v = 12;
      state increment
        entry: test_v = test_v - 1;
      state cmd
      state wait
      (default) -> test5.hand_to_270d.increment
      test5.hand_to_270d.increment -> test5.hand_to_270d.wait : after(timeToInc_1st,sec)
      test5.hand_to_270d.wait -> test5.hand_to_270d.increment [order 2] : after(timeToInc,sec)
      test5.hand_to_270d.wait -> test5.hand_to_270d.cmd [order 1] : [test_v == 6]
    state force1_to_force0
      entry: test_v = 8;
      state increment
        entry: test_v = test_v - 1;
      state cmd
        entry:
      state wait
      (default) -> test5.force1_to_force0.increment
      test5.force1_to_force0.wait -> test5.force1_to_force0.cmd [order 1] : [test_v == 2]
      test5.force1_to_force0.increment -> test5.force1_to_force0.wait : after(timeToInc_1st,sec)
      test5.force1_to_force0.wait -> test5.force1_to_force0.increment [order 2] : after(timeToInc,sec)
    state hand_dto_270d
      entry: test_v = 12;
      state increment
        entry: test_v = test_v - 1;
      state cmd
        entry:
      state wait
      (default) -> test5.hand_dto_270d.increment
      test5.hand_dto_270d.increment -> test5.hand_dto_270d.wait : after(timeToInc_1st,sec)
      test5.hand_dto_270d.wait -> test5.hand_dto_270d.increment [order 2] : after(timeToInc,sec)
      test5.hand_dto_270d.wait -> test5.hand_dto_270d.cmd [order 1] : [test_v == 2]
    state haand_to_270d
      entry: test_v = 2;
      state increment
        entry: test_v = test_v + 1;
      state cmd
        entry:
        setTN = 1;
      state wait
      (default) -> test5.haand_to_270d.increment
      test5.haand_to_270d.increment -> test5.haand_to_270d.wait : after(timeToInc_1st,sec)
      test5.haand_to_270d.wait -> test5.haand_to_270d.increment [order 2] : after(timeToInc,sec)
      test5.haand_to_270d.wait -> test5.haand_to_270d.cmd [order 1] : after(0.5,sec)[test_v == 5]
    state opcl2
      entry:
      test_command = 2;
      test_number = 9053;
    state start_test1
      entry:
      test_number = 9050;
    state opcl1
      entry:
      test_command = 3;
      test_number = 9051;
    state opcl
      entry:
      test_command = 1;
      test_number = 9052;
    state opcl3
      entry:
      test_command = 1;
      test_number = 9054;
    (default) -> test5.start_test1
    test5.start_test1 -> test5.opcl1 : [single_click == 1]
    test5.opcl2 -> test5.hand_dto_270d : [ready_stim == 1]
    test5.force1_to_force0 -> test5.opcl2 : [single_click == 1]
    test5.opcl1 -> test5.hand_to_270d : [ready_stim == 1]
    test5.opcl3 -> test5.haand_to_270d : [ready_stim == 1]
    test5.hand_to_270d.cmd -> test5.opcl : [single_click == 1]
    test5.opcl -> test5.force1_to_force0 : [ready_stim == 1]
    test5.hand_dto_270d.cmd -> test5.opcl3 : [single_click == 1]
  init_for_cont -> waitForInput1 : [testbench_cont ~= 1]
  waitForInput1 -> init_for_cont [order 1] : [testbench_cont == 1]
  waitForInput1 -> test1 [order 2] : [testbench_number == 1]
  test1 -> start : [testbench_number ~= 1]
  (default) -> init
  start -> waitForInput1 : after(0.5,sec)
  init -> start : [testbench ==1]
  waitForInput1 -> test5 [order 5] : [testbench_number == 5]
  waitForInput1 -> test4 [order 4] : [testbench_number == 4]
  waitForInput1 -> test2 [order 6] : [testbench_number == 2]
  waitForInput1 -> test3 [order 3] : [testbench_number == 3]
  test3 -> start : [testbench_number ~= 3]
  test4 -> start : [testbench_number ~= 4]
  test5 -> start : [testbench_number ~= 5]
  test2 -> start : [testbench_number ~= 2]
  data: ready_stim input; single_click input; testbench_number input; testbench input; setTN output; test_command output; test_number output; test_v output; timeToInc input; testbench_cont input; timeToInc_1st input
